simulink model "sim_4_twolink_impedance_control"  (R2021a)
settings: Solver=VariableStepAuto  StartTime=0.0  StopTime=12  MaxStep=0.01  RelTol=1e-3
values from neighbouring files (symbols this model uses):
  b1 = 0.01    [sim_params.m]    (also in sim_params_force.m)
  b2 = 0.01    [sim_params.m]    (also in sim_params_force.m)
  D = [zeros(n); eye(n)]    [control_comparison_script.m]    (also in gen_twolink_ss.m = reshape([0.0,0.0,0.0,0.0,0.0,0.0,0.0,0.0],[4,2]))
  g = 9.80665    [sim_params.m]    (also in sim_params_force.m)
  L1x = 0.3    [sim_params.m]    (also in sim_params_force.m)
  L1y = 0.050    (= 0.05)    [sim_params.m]    (also in sim_params_force.m)
  L1z = 0.05    [sim_params.m]    (also in sim_params_force.m)
  L2x = 0.15    [sim_params.m]    (also in sim_params_force.m = 0.3)
  L2y = 0.05    [sim_params.m]    (also in sim_params_force.m)
  L2z = 0.05    [sim_params.m]    (also in sim_params_force.m)
  m1 = m1*1.25    [control_comparison_script.m]    (also in sim_params.m = 2.775; sim_params_force.m = 2.775)
  m2 = m2*1.25    [control_comparison_script.m]    (also in sim_params.m = 1.3875; sim_params_force.m = 2.775)
  max_joint_torque1 = 20    [sim_params.m]    (also in sim_params_force.m)
  max_joint_torque2 = 10    [sim_params.m]    (also in sim_params_force.m = 20)
  theta1_0 = 0    [sim_params.m]    (also in sim_params_force.m = 1.57079632679)
  theta1_dot_0 = 0    [sim_params.m]    (also in sim_params_force.m)
  theta2_0 = 0    [sim_params.m]    (also in sim_params_force.m = -1.57079632679)
  theta2_dot_0 = 0    [sim_params.m]    (also in sim_params_force.m)
undefined symbols (not defined in the file or in its folder): FT_control, Impedance_no, Kdt, Ke_d, Ke_s, Kpt, Levenberg, Marquardt, Mt_inv, R_env, sigbuilder_block, W_env, X, Xenv, Y, Z
libraries: sm_lib x77, nesl_utility x58, pid_lib x6, simulink x6, robotmaniplib x3, robotcorelib x1
(part 2 of 5)

== system sim_4_twolink_impedance_control/Inverse Kinmatics/Forward Kinmatics ==
  MODEL_BUS : Inport
  Bus Creator : BusCreator  Inputs=2
  Bus Creator1 : BusCreator  Commented=on  Inputs=2
  Bus Selector : BusSelector  OutputSignals=q1,q2
  Constant : Constant  Value=L1x
  Constant1 : Constant  Value=L2x
  Demux3 : Demux  Commented=on  Outputs=3
  Forward Kinematics : MATLAB Function  TreatAsAtomicUnit=on
  Get Transform : robotmaniplib/Get Transform  Commented=on  RigidBodyTree=RR_robot  SourceBody=end_effector  TargetBody=base  SimulateUsing=Interpreted execution
  Mux2 : Mux  Commented=on  Inputs=2
  Reshape : Reshape  Commented=on
  Selector : Selector  Commented=on  InputPortWidth=16  IndexOptions=Index vector (dialog)  Indices=[13:15]  OutputSizes=1
  xy : Outport
  wires:
  Forward Kinematics/2(YE) -> Bus Creator/2  "y"
  Forward Kinematics/1(XE) -> Bus Creator/1  "x"
  Bus Selector/1 -> Mux2/1, Forward Kinematics/3(theta_1)  "<q1>"
  MODEL_BUS/1 -> Bus Selector/1
  Bus Selector/2 -> Mux2/2, Forward Kinematics/4(theta_2)  "<q2>"
  Constant/1 -> Forward Kinematics/1(L_1)
  Constant1/1 -> Forward Kinematics/2(L_2)
  Bus Creator/1 -> xy/1
  Mux2/1 -> Get Transform/1
  Get Transform/1 -> Reshape/1
  Reshape/1 -> Selector/1
  Selector/1 -> Demux3/1
  Demux3/1 -> Bus Creator1/1  "x"
  Demux3/2 -> Bus Creator1/2  "y"

== system sim_4_twolink_impedance_control/Inverse Kinmatics/IK ==
  <cmd_x> : Inport
  <cmd_y> : Inport  Port=2
  Bus Selector : BusSelector  OutputSignals=Iterations,ExitFlag
  Constant : Constant  Commented=on  Value=L1x
  Constant1 : Constant  Commented=on  Value=L2x
  Constant2 : Constant  Value=0
  Constant3 : Constant  Value=[0, 0]
  Coordinate Transformation Conversion : robotcorelib/Coordinate Transformation Conversion  InputRepresentation=Translation Vector  InputEulerSequence=ZYX  ShowTrVecInputPort=on  OutputRepresentation=Homogeneous Transformation  OutputEulerSequence=ZYX  ShowTrVecOutputPort=on  SimulateUsing=Interpreted execution
      settings: SourceProductBaseCode=RO
  Demux : Demux  Outputs=2
  IK Weights : Constant  Value=[0.1, 0.1, 0, 1, 1, 0]
  Inverse Kinematics : MATLAB Function  Commented=on  TreatAsAtomicUnit=on
  Inverse Kinematics1 : robotmaniplib/Inverse Kinematics  RigidBodyTree=RR_robot  EndEffector=end_effector  ShowInfo=on  SolverName=Levenberg-Marquardt  EnforceJointLimits=on  MaxIterations=30  MaxTime=10  GradientTolerance=1e-7  SolutionTolerance=1e-6  StepTolerance=1e-14  ErrorChangeTolerance=1e-12  UseErrorDamping=on  DampingBias=0.0025  SimulateUsing=Interpreted execution
  Mux : Mux  Inputs=3
  Scope1 : Scope
  Scope2 : Scope
  q1 : Outport
  q2 : Outport  Port=2
  wires:
  Constant1/1 -> Inverse Kinematics/4(L2)
  Constant/1 -> Inverse Kinematics/3(L1)
  <cmd_x>/1 -> Mux/1, Inverse Kinematics/1(x)
  IK Weights/1 -> Inverse Kinematics1/2
  Bus Selector/1 -> Scope2/1  "<Iterations>"
  Inverse Kinematics1/2 -> Bus Selector/1
  Coordinate Transformation Conversion/1 -> Inverse Kinematics1/1
  <cmd_y>/1 -> Inverse Kinematics/2(y), Mux/2
  Constant2/1 -> Mux/3
  Inverse Kinematics1/1 -> Demux/1
  Mux/1 -> Coordinate Transformation Conversion/1
  Bus Selector/2 -> Scope1/1  "<ExitFlag>"
  Constant3/1 -> Inverse Kinematics1/3
  Demux/2 -> q2/1  "q2_a"
  Demux/1 -> q1/1  "q1_a"

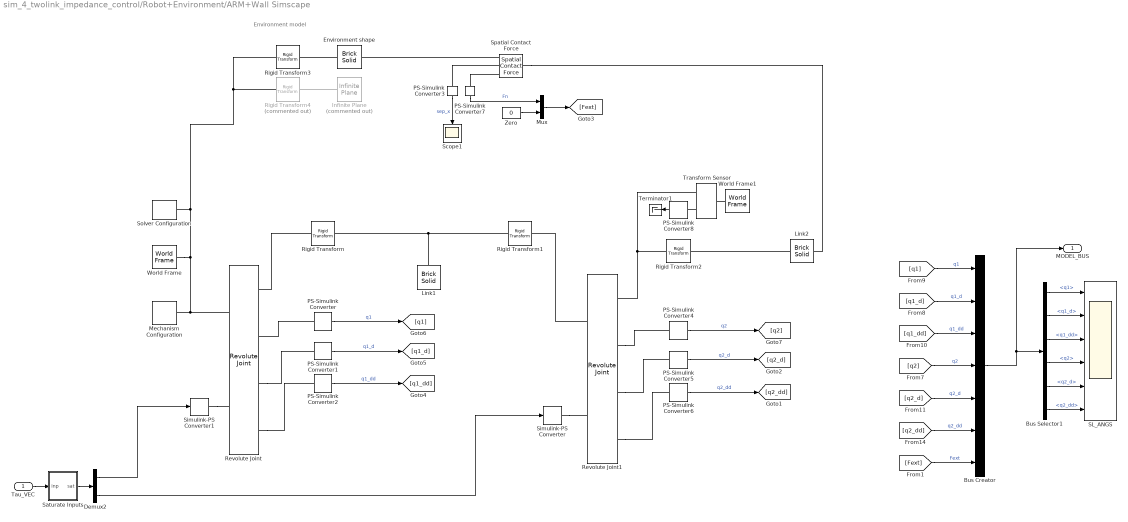
== system sim_4_twolink_impedance_control/Robot+Environment/ARM+Wall Simscape ==
  note: Environment model
  Tau_VEC : Inport
  Bus Creator : BusCreator  Inputs=7
  Bus Selector1 : BusSelector  OutputSignals=q1,q1_d,q1_dd,q2,q2_d,q2_dd
  Demux2 : Demux  Outputs=2
  Environment shape : sm_lib/Body Elements/Brick Solid  GraphicAmbientColor=[0.15 0.15 0.15 1.0]  BasedOnType=Density  BrickDimensions=[0.04 W_env 0.5]  BrickDimensionUnits=m  CenterOfMass=[0 0 0]  CenterOfMassUnits=m  GraphicDiffuseColor=[1.0 0.2 0.2]  Density=density  DensityUnits=kg/m^3  DoExposeReferenceFrame=on  GraphicEmissiveColor=[0.0 0.0 0.0 1.0]  ExportEntireGeometry=on  SerializedFrames=<Frames/>  MarkerShape=Sphere  MarkerSize=10  GraphicType=FromGeometry  InertiaType=CalculateFromGeometry  Mass=1  MassUnits=kg  MomentsOfInertia=[1 1 1]  MomentsOfInertiaUnits=kg*m^2  GraphicOpacity=1.0  ProductsOfInertia=[0 0 0]  ProductsOfInertiaUnits=kg*m^2  GraphicShininess=75  GraphicSpecularColor=[0.5 0.5 0.5 1.0]  GraphicVisPropType=SimpleVisualProperties
  Infinite Plane : sm_lib/Curves and Surfaces/Infinite Plane  Commented=on  GraphicType=Rectangle  GraphicPlaneWidth=1  GraphicPlaneWidthUnits=m  GraphicPlaneHeight=2  GraphicPlaneHeightUnits=m  GraphicVisPropType=SimpleVisualProperties  GraphicDiffuseColor=[0 0 1]  GraphicOpacity=0.25  GraphicSpecularColor=[0.5 0.5 0.5 1.0]  GraphicAmbientColor=[0.15 0.15 0.15 1.0]  GraphicEmissiveColor=[0.0 0.0 0.0 1.0]  GraphicShininess=75
  Link1 : sm_lib/Body Elements/Brick Solid  GraphicAmbientColor=[0.15 0.15 0.15 1.0]  BasedOnType=Density  BrickDimensions=[L1x L1y L1z]  BrickDimensionUnits=m  CenterOfMass=[0 0 0]  CenterOfMassUnits=m  GraphicDiffuseColor=[0.8 0.8 1.0]  Density=density  DensityUnits=kg/m^3  DoExposeReferenceFrame=on  GraphicEmissiveColor=[0.0 0.0 0.0 1.0]  ExportEntireGeometry=off  SerializedFrames=<Frames/>  MarkerShape=Sphere  MarkerSize=10  GraphicType=FromGeometry  InertiaType=CalculateFromGeometry  Mass=1  MassUnits=kg  MomentsOfInertia=[1 1 1]  MomentsOfInertiaUnits=kg*m^2  GraphicOpacity=1.0  ProductsOfInertia=[0 0 0]  ProductsOfInertiaUnits=kg*m^2  GraphicShininess=75  GraphicSpecularColor=[0.5 0.5 0.5 1.0]  GraphicVisPropType=SimpleVisualProperties
  Link2 : sm_lib/Body Elements/Brick Solid  GraphicAmbientColor=[0.15 0.15 0.15 1.0]  BasedOnType=Density  BrickDimensions=[L2x L2y L2z]  BrickDimensionUnits=m  CenterOfMass=[0 0 0]  CenterOfMassUnits=m  GraphicDiffuseColor=[1.0 0.6 1.0]  Density=density  DensityUnits=kg/m^3  DoExposeReferenceFrame=on  GraphicEmissiveColor=[0.0 0.0 0.0 1.0]  ExportEntireGeometry=on  SerializedFrames=<Frames/>  MarkerShape=Sphere  MarkerSize=10  GraphicType=FromGeometry  InertiaType=CalculateFromGeometry  Mass=1  MassUnits=kg  MomentsOfInertia=[1 1 1]  MomentsOfInertiaUnits=kg*m^2  GraphicOpacity=1.0  ProductsOfInertia=[0 0 0]  ProductsOfInertiaUnits=kg*m^2  GraphicShininess=75  GraphicSpecularColor=[0.5 0.5 0.5 1.0]  GraphicVisPropType=SimpleVisualProperties
  Mechanism Configuration : sm_lib/Utilities/Mechanism Configuration  UniformGravity=Constant  GravityVector=[0 -g 0 ]  GravityVectorUnits=m/s^2  GravityUnits=m/s^2  LinearizationDelta=1e-4  JointModeTransitionNonlinearIterations=2
  Mux : Mux  Inputs=2
  PS-Simulink Converter : nesl_utility/PS-Simulink Converter  PhysicalDomain=network_engine_domain  SubClassName=ps_output  LeftPortType=input  RightPortType=output  PseudoPeriodic=off  Frequencies=[]  Unit=rad  AffineConversion=off
      settings: SourceProductBaseCode=PW,SS
  PS-Simulink Converter1 : nesl_utility/PS-Simulink Converter  PhysicalDomain=network_engine_domain  SubClassName=ps_output  LeftPortType=input  RightPortType=output  PseudoPeriodic=off  Frequencies=[]  Unit=rad/s  AffineConversion=off
      settings: SourceProductBaseCode=PW,SS
  PS-Simulink Converter2 : nesl_utility/PS-Simulink Converter  PhysicalDomain=network_engine_domain  SubClassName=ps_output  LeftPortType=input  RightPortType=output  PseudoPeriodic=off  Frequencies=[]  Unit=rad/s^2  AffineConversion=off
      settings: SourceProductBaseCode=PW,SS
  PS-Simulink Converter3 : nesl_utility/PS-Simulink Converter  PhysicalDomain=network_engine_domain  SubClassName=ps_output  LeftPortType=input  RightPortType=output  PseudoPeriodic=off  Frequencies=[]  Unit=inherit  AffineConversion=off
      settings: SourceProductBaseCode=PW,SS
  PS-Simulink Converter4 : nesl_utility/PS-Simulink Converter  PhysicalDomain=network_engine_domain  SubClassName=ps_output  LeftPortType=input  RightPortType=output  PseudoPeriodic=off  Frequencies=[]  Unit=rad  AffineConversion=off
      settings: SourceProductBaseCode=PW,SS
  PS-Simulink Converter5 : nesl_utility/PS-Simulink Converter  PhysicalDomain=network_engine_domain  SubClassName=ps_output  LeftPortType=input  RightPortType=output  PseudoPeriodic=off  Frequencies=[]  Unit=rad/s  AffineConversion=off
      settings: SourceProductBaseCode=PW,SS
  PS-Simulink Converter6 : nesl_utility/PS-Simulink Converter  PhysicalDomain=network_engine_domain  SubClassName=ps_output  LeftPortType=input  RightPortType=output  PseudoPeriodic=off  Frequencies=[]  Unit=rad/s^2  AffineConversion=off
      settings: SourceProductBaseCode=PW,SS
  PS-Simulink Converter7 : nesl_utility/PS-Simulink Converter  PhysicalDomain=network_engine_domain  SubClassName=ps_output  LeftPortType=input  RightPortType=output  PseudoPeriodic=off  Frequencies=[]  Unit=inherit  AffineConversion=off
      settings: SourceProductBaseCode=PW,SS
  PS-Simulink Converter8 : nesl_utility/PS-Simulink Converter  PhysicalDomain=network_engine_domain  SubClassName=ps_output  LeftPortType=input  RightPortType=output  PseudoPeriodic=off  Frequencies=[]  Unit=1  AffineConversion=off
      settings: SourceProductBaseCode=PW,SS
  Revolute Joint : sm_lib/Joints/Revolute Joint  JointMode=Normal  SenseConstraintForce=off  SenseConstraintForceX=off  SenseConstraintForceY=off  SenseConstraintForceZ=off  SenseConstraintTorque=off  SenseConstraintTorqueX=off  SenseConstraintTorqueY=off  SenseConstraintTorqueZ=off  SenseTotalForce=off  SenseTotalForceX=off  SenseTotalForceY=off  SenseTotalForceZ=off  SenseTotalTorque=off  SenseTotalTorqueX=off  SenseTotalTorqueY=off  SenseTotalTorqueZ=off  CompositeWrenchDir=BaseOnFollower  CompositeWrenchFrame=BaseFrame  EquilibriumPosition=0  EquilibriumPositionUnits=deg  SpringStiffness=0  SpringStiffnessUnits=N*m/deg  DampingCoefficient=b1  DampingCoefficientUnits=N*m/(rad/s)  TorqueActuationMode=InputTorque  MotionActuationMode=ComputedMotion  SensePosition=on  SenseVelocity=on  SenseAcceleration=on  SenseTorqueForce=off  SenseLowerLimitTorqueForce=off  SenseUpperLimitTorqueForce=off  LowerLimitSpecify=off  LowerLimitBound=-90  LowerLimitBoundUnits=deg  LowerLimitStiffness=1e4  LowerLimitStiffnessUnits=N*m/deg  LowerLimitDamping=10  LowerLimitDampingUnits=N*m/(deg/s)  LowerLimitTransitionRegionWidth=0.1  LowerLimitTransitionRegionWidthUnits=deg  UpperLimitSpecify=off  UpperLimitBound=90  UpperLimitBoundUnits=deg  UpperLimitStiffness=1e4  UpperLimitStiffnessUnits=N*m/deg  UpperLimitDamping=10  UpperLimitDampingUnits=N*m/(deg/s)  UpperLimitTransitionRegionWidth=0.1  UpperLimitTransitionRegionWidthUnits=deg  PositionTargetSpecify=on  PositionTargetPriority=Low  PositionTargetValue=theta1_0  PositionTargetValueUnits=rad  VelocityTargetSpecify=on  VelocityTargetPriority=High  VelocityTargetValue=theta1_dot_0  VelocityTargetValueUnits=rad/s
      settings: AttributesFormatString=|
      | %<DampingCoefficient>
      | %<PositionTargetValue>
      | %<VelocityTargetValue>
  Revolute Joint1 : sm_lib/Joints/Revolute Joint  JointMode=Normal  SenseConstraintForce=off  SenseConstraintForceX=off  SenseConstraintForceY=off  SenseConstraintForceZ=off  SenseConstraintTorque=off  SenseConstraintTorqueX=off  SenseConstraintTorqueY=off  SenseConstraintTorqueZ=off  SenseTotalForce=off  SenseTotalForceX=off  SenseTotalForceY=off  SenseTotalForceZ=off  SenseTotalTorque=off  SenseTotalTorqueX=off  SenseTotalTorqueY=off  SenseTotalTorqueZ=off  CompositeWrenchDir=BaseOnFollower  CompositeWrenchFrame=FollowerFrame  EquilibriumPosition=0  EquilibriumPositionUnits=deg  SpringStiffness=0  SpringStiffnessUnits=N*m/deg  DampingCoefficient=b2  DampingCoefficientUnits=N*m/(rad/s)  TorqueActuationMode=InputTorque  MotionActuationMode=ComputedMotion  SensePosition=on  SenseVelocity=on  SenseAcceleration=on  SenseTorqueForce=off  SenseLowerLimitTorqueForce=off  SenseUpperLimitTorqueForce=off  LowerLimitSpecify=off  LowerLimitBound=-90  LowerLimitBoundUnits=deg  LowerLimitStiffness=1e4  LowerLimitStiffnessUnits=N*m/deg  LowerLimitDamping=10  LowerLimitDampingUnits=N*m/(deg/s)  LowerLimitTransitionRegionWidth=0.1  LowerLimitTransitionRegionWidthUnits=deg  UpperLimitSpecify=off  UpperLimitBound=90  UpperLimitBoundUnits=deg  UpperLimitStiffness=1e4  UpperLimitStiffnessUnits=N*m/deg  UpperLimitDamping=10  UpperLimitDampingUnits=N*m/(deg/s)  UpperLimitTransitionRegionWidth=0.1  UpperLimitTransitionRegionWidthUnits=deg  PositionTargetSpecify=on  PositionTargetPriority=Low  PositionTargetValue=theta2_0  PositionTargetValueUnits=rad  VelocityTargetSpecify=on  VelocityTargetPriority=High  VelocityTargetValue=theta2_dot_0  VelocityTargetValueUnits=rad/s
      settings: AttributesFormatString=|
      | %<DampingCoefficient>
      | %<PositionTargetValue>
      | %<VelocityTargetValue>
  Rigid Transform : sm_lib/Frames and Transforms/Rigid Transform  TranslationMethod=StandardAxis  TranslationStandardOffset=L1x/2  TranslationLengthUnit=m  TranslationStandardAxis=+X  TranslationCartesianOffset=[0 0 0]  TranslationROffset=0  TranslationROffsetUnits=m  TranslationZOffset=0  TranslationZOffsetUnits=m  TranslationThetaOffset=0  TranslationThetaOffsetUnits=deg  RotationMethod=None  RotationAngleUnits=deg  RotationStandardAxis=+Z  RotationAngle=0.0  RotationArbitraryAxis=[0 0 1]  FollAlignAxisA=+X  BaseAlignAxisA=+Y  FollAlignAxisB=+Y  BaseAlignAxisB=+Z  RotationSequenceAxes=FollowerAxes  RotationSequence=XYX  RotationSequenceAngles=[0 0 0]  RotationSequenceAnglesUnits=deg  RotationMatrix=[1 0 0; 0 1 0; 0 0 1]
  Rigid Transform1 : sm_lib/Frames and Transforms/Rigid Transform  TranslationMethod=StandardAxis  TranslationStandardOffset=L1x/2  TranslationLengthUnit=m  TranslationStandardAxis=+X  TranslationCartesianOffset=[0 0 0]  TranslationROffset=0  TranslationROffsetUnits=m  TranslationZOffset=0  TranslationZOffsetUnits=m  TranslationThetaOffset=0  TranslationThetaOffsetUnits=deg  RotationMethod=None  RotationAngleUnits=deg  RotationStandardAxis=+Z  RotationAngle=0.0  RotationArbitraryAxis=[0 0 1]  FollAlignAxisA=+X  BaseAlignAxisA=+Y  FollAlignAxisB=+Y  BaseAlignAxisB=+Z  RotationSequenceAxes=FollowerAxes  RotationSequence=XYX  RotationSequenceAngles=[0 0 0]  RotationSequenceAnglesUnits=deg  RotationMatrix=[1 0 0; 0 1 0; 0 0 1]
  Rigid Transform2 : sm_lib/Frames and Transforms/Rigid Transform  TranslationMethod=StandardAxis  TranslationStandardOffset=L2x/2  TranslationLengthUnit=m  TranslationStandardAxis=+X  TranslationCartesianOffset=[0 0 0]  TranslationROffset=0  TranslationROffsetUnits=m  TranslationZOffset=0  TranslationZOffsetUnits=m  TranslationThetaOffset=0  TranslationThetaOffsetUnits=deg  RotationMethod=None  RotationAngleUnits=deg  RotationStandardAxis=+Z  RotationAngle=0.0  RotationArbitraryAxis=[0 0 1]  FollAlignAxisA=+X  BaseAlignAxisA=+Y  FollAlignAxisB=+Y  BaseAlignAxisB=+Z  RotationSequenceAxes=FollowerAxes  RotationSequence=XYX  RotationSequenceAngles=[0 0 0]  RotationSequenceAnglesUnits=deg  RotationMatrix=[1 0 0; 0 1 0; 0 0 1]
  Rigid Transform3 : sm_lib/Frames and Transforms/Rigid Transform  TranslationMethod=StandardAxis  TranslationStandardOffset=Xenv+(L2y/2)-(1e-3)  TranslationLengthUnit=m  TranslationStandardAxis=+X  TranslationCartesianOffset=[0 0 0]  TranslationROffset=0  TranslationROffsetUnits=m  TranslationZOffset=0  TranslationZOffsetUnits=m  TranslationThetaOffset=0  TranslationThetaOffsetUnits=deg  RotationMethod=None  RotationAngleUnits=deg  RotationStandardAxis=+Z  RotationAngle=0.0  RotationArbitraryAxis=[0 0 1]  FollAlignAxisA=+X  BaseAlignAxisA=+Y  FollAlignAxisB=+Y  BaseAlignAxisB=+Z  RotationSequenceAxes=FollowerAxes  RotationSequence=XYX  RotationSequenceAngles=[0 0 0]  RotationSequenceAnglesUnits=deg  RotationMatrix=[1 0 0; 0 1 0; 0 0 1]
  Rigid Transform4 : sm_lib/Frames and Transforms/Rigid Transform  Commented=on  TranslationMethod=StandardAxis  TranslationStandardOffset=1  TranslationLengthUnit=m  TranslationStandardAxis=+X  TranslationCartesianOffset=[0 0 0]  TranslationROffset=0  TranslationROffsetUnits=m  TranslationZOffset=0  TranslationZOffsetUnits=m  TranslationThetaOffset=0  TranslationThetaOffsetUnits=deg  RotationMethod=AlignedAxes  RotationAngleUnits=deg  RotationStandardAxis=+Z  RotationAngle=0.0  RotationArbitraryAxis=[0 0 1]  FollAlignAxisA=+Z  BaseAlignAxisA=+X  FollAlignAxisB=+X  BaseAlignAxisB=+Z  RotationSequenceAxes=FollowerAxes  RotationSequence=XYX  RotationSequenceAngles=[0 0 0]  RotationSequenceAnglesUnits=deg  RotationMatrix=[1 0 0; 0 1 0; 0 0 1]
  SL_ANGS : Scope  NumInputPorts=6
  Saturate Inputs : Subsystem
  Scope1 : Scope
  Simulink-PS Converter : nesl_utility/Simulink-PS Converter  PhysicalDomain=network_engine_domain  SubClassName=ps_input  LeftPortType=input  RightPortType=output  PseudoPeriodic=off  Frequencies=[]  NoiseDistribution=none  NoiseParameters=[]  Unit=N*m  AffineConversion=off  FilteringAndDerivatives=zero  SimscapeFilterOrder=1  InputFilterTimeConstant=0.001  UdotUserProvided=1
      settings: SourceProductBaseCode=PW,SS
  Simulink-PS Converter1 : nesl_utility/Simulink-PS Converter  PhysicalDomain=network_engine_domain  SubClassName=ps_input  LeftPortType=input  RightPortType=output  PseudoPeriodic=off  Frequencies=[]  NoiseDistribution=none  NoiseParameters=[]  Unit=N*m  AffineConversion=off  FilteringAndDerivatives=zero  SimscapeFilterOrder=1  InputFilterTimeConstant=0.001  UdotUserProvided=1
      settings: SourceProductBaseCode=PW,SS
  Solver Configuration : nesl_utility/Solver Configuration  PhysicalDomain=network_engine_domain  SubClassName=solver  LeftPortType=input  RightPortType=generic  Tones=[]  Harmonics=[]  SimulateNoise=off  Profile=off  UseLocalSampling=off  EnableSwitchedLinearOptims=on  FrequencyDomain=off  UseCCode=off  RelTol=0.001  AbsTol=1e-06  MinStep=1e-09  ToWorkspace=off  RevertToSquareIcSolve=off  NumHomotopyIterations=100  PhasorMode=off  PhasorModeNumHarmonics=1  DoDC=off  ResidualTolerance=1e-09  UseLocalSolver=off  LocalSolverChoice=NE_TRAPEZOIDAL_ADVANCER  LocalSolverSampleTime=0.01  DoFixedCost=off  MaxNonlinIter=3  MaxModeIter=2  ComputeImpulses=off  ImpulseIterations=2  LinearAlgebra=Sparse  EquationFormulation=NE_TIME_EF  DelaysMemoryBudget=1024  AutomaticFiltering=off  FilteringTimeConstant=0.001  PartitionStorageMethod=AS_NEEDED  PartitionMemoryBudget=1024  PartitionMethod=FAST
      settings: SourceProductBaseCode=PW,SS
  Spatial Contact Force : sm_lib/Forces and Torques/Spatial Contact Force  CoefficientOfDynamicFriction=0.3  CoefficientOfStaticFriction=0.5  SenseContactBaseRotation=off  SenseContactBaseTranslation=off  NormalDamping=Ke_d  NormalDampingUnits=N/(m/s)  SenseContactFollowerRotation=off  SenseContactFollowerTranslation=off  SenseContactSignal=off  NormalStiffness=Ke_s  NormalStiffnessUnits=N/m  FrictionalCriticalVelocity=1e-3  FrictionalCriticalVelocityUnits=m/s  ZeroCrossDetectContactStartAndEnd=off  FrictionType=None  SenseFrictionalForceMagnitude=off  SenseNormalForceMagnitude=on  NormalForceType=SmoothSpringDamper  SenseNormalVelocity=off  SenseSeparationDistance=on  SenseTangentialVelocity=off  SenseTangentialVelocityMagnitude=off  NormalTransitionRegionWidth=1e-3  NormalTransitionRegionWidthUnits=m
  Terminator1 : Terminator
  Transform Sensor : sm_lib/Frames and Transforms/Transform Sensor  MeasurementFrame=World  SenseAngle=off  SenseAxis=off  SenseAngle1=off  SenseAngle2=off  SenseAngle3=off  SenseQ=off  SenseR=on  SenseOmegaX=off  SenseOmegaY=off  SenseOmegaZ=off  SenseOmega1=off  SenseOmega2=off  SenseOmega3=off  SenseQDot=off  SenseRDot=off  SenseAlphaX=off  SenseAlphaY=off  SenseAlphaZ=off  SenseAlpha1=off  SenseAlpha2=off  SenseAlpha3=off  SenseQDDot=off  SenseRDDot=off  SenseX=off  SenseY=off  SenseZ=off  SenseRad=off  SenseAzim=off  SenseDist=off  SenseInc=off  SenseXDot=off  SenseYDot=off  SenseZDot=off  SenseRadDot=off  SenseAzimDot=off  SenseDistDot=off  SenseIncDot=off  SenseXDDot=off  SenseYDDot=off  SenseZDDot=off  SenseRadDDot=off  SenseAzimDDot=off  SenseDistDDot=off  SenseIncDDot=off
  World Frame : sm_lib/Frames and Transforms/World Frame
  World Frame1 : sm_lib/Frames and Transforms/World Frame
  Zero : Constant  Value=0  OutDataTypeStr=Inherit: Inherit via back propagation
  MODEL_BUS : Outport
  wires:
  PS-Simulink Converter/1 -> [q1]  "q1"
  PS-Simulink Converter2/1 -> [q1_dd]  "q1_dd"
  PS-Simulink Converter1/1 -> [q1_d]  "q1_d"
  Bus Creator/1 -> Bus Selector1/1, MODEL_BUS/1
  PS-Simulink Converter4/1 -> [q2]  "q2"
  PS-Simulink Converter6/1 -> [q2_dd]  "q2_dd"
  PS-Simulink Converter5/1 -> [q2_d]  "q2_d"
  Tau_VEC/1 -> Saturate Inputs/1(inp)
  Demux2/1 -> Simulink-PS Converter1/1
  Demux2/2 -> Simulink-PS Converter/1
  Bus Selector1/2 -> SL_ANGS/2  "<q1_d>"
  Bus Selector1/5 -> SL_ANGS/5  "<q2_d>"
  Bus Selector1/6 -> SL_ANGS/6  "<q2_dd>"
  Bus Selector1/1 -> SL_ANGS/1  "<q1>"
  Bus Selector1/3 -> SL_ANGS/3  "<q1_dd>"
  [q1_dd] -> Bus Creator/3  "q1_dd"
  [q1] -> Bus Creator/1  "q1"
  [q2] -> Bus Creator/4  "q2"
  [q2_d] -> Bus Creator/5  "q2_d"
  [q1_d] -> Bus Creator/2  "q1_d"
  [q2_dd] -> Bus Creator/6  "q2_dd"
  Bus Selector1/4 -> SL_ANGS/4  "<q2>"
  PS-Simulink Converter8/1 -> Terminator1/1
  Saturate Inputs/1(sat) -> Demux2/1
  PS-Simulink Converter7/1 -> Mux/1  "Fn"
  PS-Simulink Converter3/1 -> Scope1/1  "sep_x"
  Mux/1 -> [Fext]
  Zero/1 -> Mux/2
  [Fext] -> Bus Creator/7  "Fext"
  connections:
  World Frame/RConn1 -- Revolute Joint/LConn1 -- Mechanism Configuration/RConn1 -- Rigid Transform4/LConn1 -- Rigid Transform3/LConn1 -- Solver Configuration/RConn1
  Rigid Transform1/LConn1 -- Link1/RConn1 -- Rigid Transform/RConn1
  Revolute Joint/RConn3 -- PS-Simulink Converter1/LConn1
  Revolute Joint/RConn4 -- PS-Simulink Converter2/LConn1
  Rigid Transform/LConn1 -- Revolute Joint/RConn1
  PS-Simulink Converter/LConn1 -- Revolute Joint/RConn2
  Revolute Joint1/LConn1 -- Rigid Transform1/RConn1
  Revolute Joint1/RConn3 -- PS-Simulink Converter5/LConn1
  Revolute Joint1/RConn2 -- PS-Simulink Converter4/LConn1
  Revolute Joint1/RConn4 -- PS-Simulink Converter6/LConn1
  Link2/RConn1 -- Rigid Transform2/RConn1
  Rigid Transform2/LConn1 -- Transform Sensor/RConn1 -- Revolute Joint1/RConn1
  World Frame1/RConn1 -- Transform Sensor/LConn1
  PS-Simulink Converter8/LConn1 -- Transform Sensor/RConn2
  Simulink-PS Converter/RConn1 -- Revolute Joint1/LConn2
  Simulink-PS Converter1/RConn1 -- Revolute Joint/LConn2
  Environment shape/RConn1 -- Rigid Transform3/RConn1
  Infinite Plane/LConn1 -- Rigid Transform4/RConn1
  Spatial Contact Force/LConn1 -- Link2/LConn1
  Spatial Contact Force/RConn1 -- Environment shape/LConn1
  PS-Simulink Converter3/LConn1 -- Spatial Contact Force/RConn2
  Spatial Contact Force/RConn3 -- PS-Simulink Converter7/LConn1

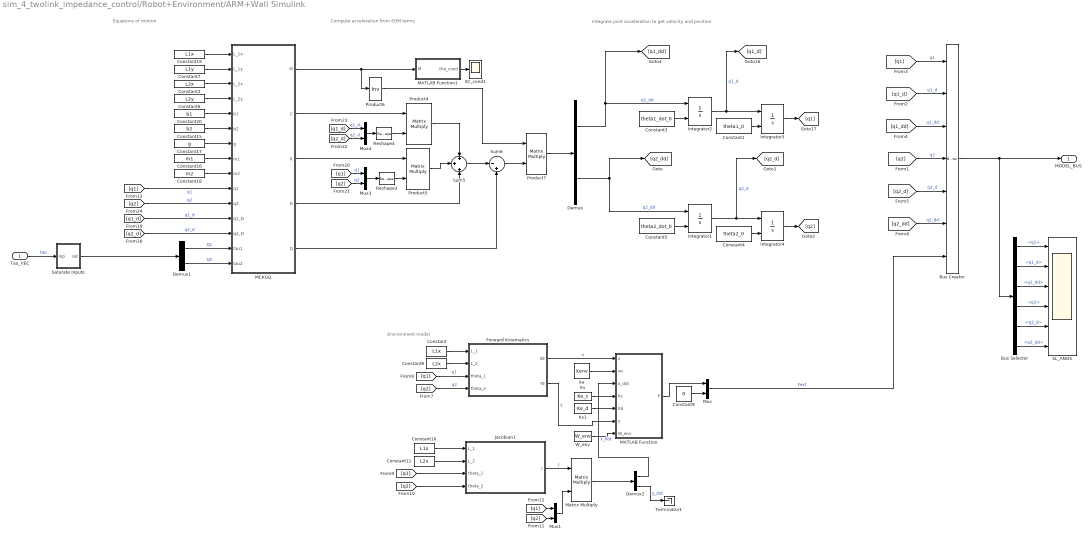
== system sim_4_twolink_impedance_control/Robot+Environment/ARM+Wall Simulink ==
  note: Integrate joint acceleration to get velocity and position
  note: Compute acceleration from EOM terms
  note: Equations of motion
  note: Environment model
  Tau_VEC : Inport
  Bus Creator : BusCreator  Inputs=7
  Bus Selector : BusSelector  OutputSignals=q1,q1_d,q1_dd,q2,q2_d,q2_dd
  Constant : Constant  Value=L1x
  Constant1 : Constant  Value=theta1_0
  Constant10 : Constant  Value=L1x
  Constant11 : Constant  Value=L2x
  Constant15 : Constant  Value=b2
  Constant16 : Constant  Value=m1
  Constant17 : Constant  Value=g
  Constant18 : Constant  Value=m2
  Constant19 : Constant  Value=L1x
  Constant2 : Constant  Value=L2x
  Constant20 : Constant  Value=b1
  Constant3 : Constant  Value=theta1_dot_0
  Constant4 : Constant  Value=theta2_0
  Constant5 : Constant  Value=theta2_dot_0
  Constant6 : Constant  Value=L2y
  Constant7 : Constant  Value=L1y
  Constant8 : Constant  Value=L2x
  Constant9 : Constant  Value=0
  Demux : Demux  Outputs=2
  Demux1 : Demux  Outputs=2
  Demux2 : Demux  Outputs=2
  Forward Kinematics : MATLAB Function  TreatAsAtomicUnit=on
  Integrator{1..4} (4 alike) : Integrator  InitialConditionSource=external
  Jacobian1 : MATLAB Function  TreatAsAtomicUnit=on
  Ks : Constant  Value=Ke_s
  Ks1 : Constant  Value=Ke_d
  MATLAB Function : MATLAB Function  TreatAsAtomicUnit=on
  MATLAB Function1 : MATLAB Function  TreatAsAtomicUnit=on
  MCKGQ : MATLAB Function  TreatAsAtomicUnit=on
  Matrix Multiply : Product  Multiplication=Matrix(*)
  Mux{,1,3..4} (4 alike) : Mux  Inputs=2
  Product4 : Product  Multiplication=Matrix(*)
  Product5 : Product  Multiplication=Matrix(*)
  Product6 : Product  Inputs=/  Multiplication=Matrix(*)
  Product7 : Product  Multiplication=Matrix(*)
  Reshape3 : Reshape  OutputDimensionality=Column vector (2-D)
  Reshape4 : Reshape  OutputDimensionality=Column vector (2-D)
  SC_cond1 : Scope
  SL_ANGS : Scope  NumInputPorts=6
  Saturate Inputs : Subsystem
  Sum5 : Sum  Inputs=+|+|+
  Sum6 : Sum  Inputs=|-+
  Terminator1 : Terminator
  W_env : Constant  Value=W_env
  Xe : Constant  Value=Xenv
  MODEL_BUS : Outport
  wires:
  Bus Creator/1 -> MODEL_BUS/1, Bus Selector/1
  Bus Selector/2 -> SL_ANGS/2  "<q1_d>"
  Bus Selector/3 -> SL_ANGS/3  "<q1_dd>"
  Bus Selector/1 -> SL_ANGS/1  "<q1>"
  Bus Selector/4 -> SL_ANGS/4  "<q2>"
  Bus Selector/6 -> SL_ANGS/6  "<q2_dd>"
  Integrator3/1 -> [q1]
  Integrator2/1 -> [q1_d], Integrator3/1  "q1_d"
  Constant3/1 -> Integrator2/2
  Constant1/1 -> Integrator3/2
  Integrator1/1 -> [q2_d], Integrator4/1  "q2_d"
  Constant4/1 -> Integrator4/2
  Integrator4/1 -> [q2]
  Constant5/1 -> Integrator1/2
  [q1_d] -> Bus Creator/2  "q1_d"
  [q2_d] -> Bus Creator/5  "q2_d"
  [q2] -> Bus Creator/4  "q2"
  [q2_dd] -> Bus Creator/6  "q2_dd"
  [q1] -> Bus Creator/1  "q1"
  [q1_dd] -> Bus Creator/3  "q1_dd"
  Demux/1 -> [q1_dd], Integrator2/1  "q1_dd"
  Demux/2 -> [q2_dd], Integrator1/1  "q2_dd"
  MCKGQ/5(Q) -> Sum6/2
  [q1] -> Mux3/1  "q1"
  Sum6/1 -> Product7/2
  [q2] -> Mux3/2  "q2"
  Sum5/1 -> Sum6/1
  Product4/1 -> Sum5/1
  Constant18/1 -> MCKGQ/9(m2)
  Product5/1 -> Sum5/2
  Demux1/2 -> MCKGQ/15(tau2)  "Q2"
  MCKGQ/3(K) -> Product5/1
  MATLAB Function1/1(the_cond) -> SC_cond1/1
  Product6/1 -> Product7/1
  Constant20/1 -> MCKGQ/5(b1)
  Reshape3/1 -> Product5/2
  [q1] -> MCKGQ/10(q1)  "q1"
  Constant6/1 -> MCKGQ/4(L_2y)
  MCKGQ/4(G) -> Sum5/3
  Constant15/1 -> MCKGQ/6(b2)
  [q1_d] -> MCKGQ/12(q1_D)  "q1_d"
  Constant2/1 -> MCKGQ/3(L_2x)
  Constant19/1 -> MCKGQ/1(L_1x)
  Constant7/1 -> MCKGQ/2(L_1y)
  MCKGQ/2(C) -> Product4/1
  [q1_d] -> Mux4/1  "q1_d"
  Mux3/1 -> Reshape3/1
  Reshape4/1 -> Product4/2
  [q2_d] -> MCKGQ/13(q2_D)  "q2_d"
  [q2_d] -> Mux4/2  "q2_d"
  Demux1/1 -> MCKGQ/14(tau1)  "Q1"
  MCKGQ/1(M) -> MATLAB Function1/1(M), Product6/1
  Mux4/1 -> Reshape4/1
  [q2] -> MCKGQ/11(q2)  "q2"
  Constant17/1 -> MCKGQ/7(g)
  Constant16/1 -> MCKGQ/8(m1)
  Product7/1 -> Demux/1
  Bus Selector/5 -> SL_ANGS/5  "<q2_d>"
  Tau_VEC/1 -> Saturate Inputs/1(inp)  "tau"
  Saturate Inputs/1(sat) -> Demux1/1
  Constant/1 -> Forward Kinematics/1(L_1)
  Forward Kinematics/1(XE) -> MATLAB Function/1(x)  "x"
  Forward Kinematics/2(YE) -> MATLAB Function/6(y)  "y"
  Constant8/1 -> Forward Kinematics/2(L_2)
  Xe/1 -> MATLAB Function/2(xe)
  Ks/1 -> MATLAB Function/4(Ks)
  Constant9/1 -> Mux/2
  Mux/1 -> Bus Creator/7  "Fext"
  [q1] -> Forward Kinematics/3(theta_1)  "q1"
  [q2] -> Forward Kinematics/4(theta_2)  "q2"
  Demux2/1 -> MATLAB Function/3(x_dot)  "x_dot"
  Mux1/1 -> Matrix Multiply/2
  [q1] -> Jacobian1/3(theta_1)
  Jacobian1/1(J) -> Matrix Multiply/1  "J"
  Constant11/1 -> Jacobian1/2(L_2)
  [q2] -> Jacobian1/4(theta_2)
  Constant10/1 -> Jacobian1/1(L_1)
  Matrix Multiply/1 -> Demux2/1
  [q2] -> Mux1/2
  [q1] -> Mux1/1
  Demux2/2 -> Terminator1/1  "y_dot"
  MATLAB Function/1(F) -> Mux/1
  Ks1/1 -> MATLAB Function/5(Kd)
  W_env/1 -> MATLAB Function/7(W_env)
